simulink model "volo_radio_controller"  (Simulink 8.0)
settings: Solver=ode45  SolverMode=SingleTasking  StartTime=0.0  StopTime=1000  RelTol=1e-3
InitFcn:
  | volo_radio_controller_init
values from neighbouring files (symbols this model uses):
  cFI = fi(cMult, 1, 13, 11)    [volo_radio_controller_init.m]
  gFI = fi(gain, 1, 13, 11)    [volo_radio_controller_init.m]
  sFI = fi(sMult, 1, 13, 11)    [volo_radio_controller_init.m]
undefined symbols (not defined in the file or in its folder): gcbh, xlBlockLoadCallback, xlGetNormalizedPeriod, xlipgetpartsetting
libraries: xbsIndex_r4 x380, xbsEDKLib_r4 x1
(part 1 of 5)
settings Model: Creator=naren  LastModifiedBy=rng
settings DataIOCC: SignalLoggingSaveFormat=ModelDataLogs
settings DebuggingCC: FcnCallInpInsideContextMsg=UseLocalSettings
settings GRTTargetCC: CombineOutputUpdateFcns=off  GRTInterface=on

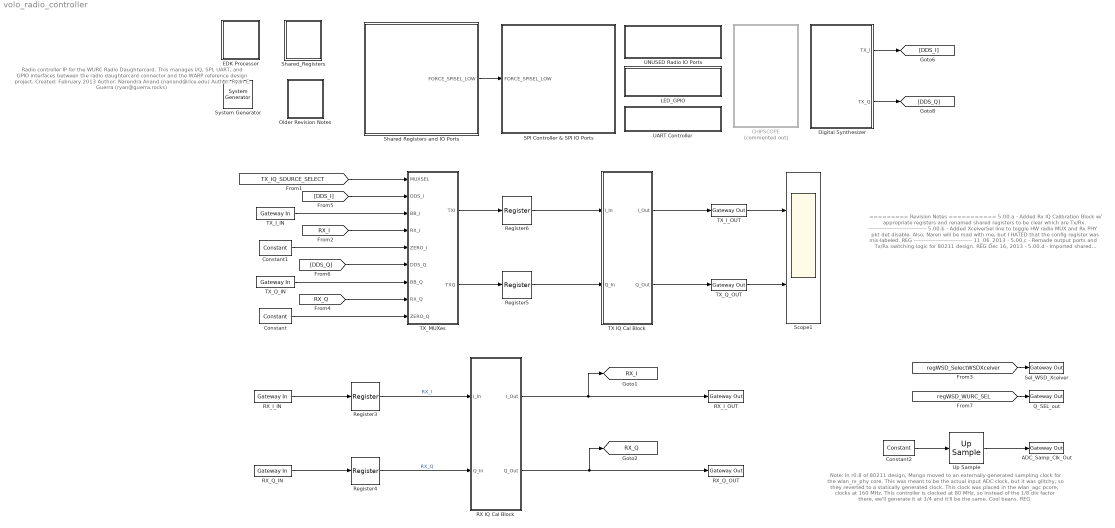
== system volo_radio_controller ==
  note: Note: in r0.8 of 80211 design, Mango moved to an externally-generated sampling clock for the wlan_rx_phy
      | core. This was meant to be the actual input ADC clock, but it was glitchy, so they reverted to a statically generated clock.
      | This clock was placed in the wlan_agc pcore, clocks at 160 MHz. This controller is clocked at 80 MHz, so instead of the 1/8
      | div factor there, we'll generate it at 1/4 and it'll be the same. Cool beans. REG
  note: Radio controller IP for the WURC Radio Daughtercard.
      | This manages I/Q, SPI, UART, and GPIO interfaces
      | between the radio daughtercard connector and the
      | WARP reference design project.
      |
      | Created: February 2013
      | Author: Narendra Anand (nanand@rice.edu)
      | Author: Ryan E. Guerra (ryan@guerra.rocks)
  note: ========= Revision Notes ===========
      | 5.00.a - Added Rx IQ Calibration Block w/ appropriate registers and renamed shared
      | registers to be clear which are Tx/Rx.
      | -----------------------------------
      | 5.00.b - Added XceiverSel line to toggle HW radio MUX and Rx PHY pkt det disable.
      | Also, Naren will be mad with me, but I HATED that the config register was mis-labeled. REG
      | -----------------------------------
      | 11_06_2013 - 5.00.c - Remade output ports and Tx/Rx switching logic for 80211 design. REG
      | Dec 16, 2013 - 5.00.d - Imported shared registers from Tx/Rx FIR to save on AXI Slave slots REG
      | Jan 15, 2014 - 5.00.e - Removed filter stuff and cleaned up for 802.11 Rev0.7 REG
      | Jan 17, 2014 - 5.00.f - removed extra ports to avoid confusion. Better to add than take away REG
      | Feb 13, 2014 - 5.00.g - added ADC_SAMP_CLK_OUT port for compatibility with rev 0.8 design REG
      | April 22, 2014 - 5.00.h - Changed DDS synthesizer tp fixed Sysgen core for better frequency response
      | AND removed the corresponding DDS registers (phaseInc and ddsOutputReset) NA
      | April 29, 2014 - 5.00.i - Previous version had some EDK register screwup, fixed now.  NA
      | April 30, 2014 - 5.00.j - Added taylor series correction setting to dds compiler, maximized DSP
      | utilization and set goal to speed.
      | May 23, 2014 - 5.08.k - WOW! EDK Processor was creating duplicate register offset addresses.
      | This was the problem that was borking everything. NOTE: it is still not fixed, but we have gone and
      | hand-edited the MPD file with unique, non-overlapping offsets for the To/From registers. REG
      | May 23, 2014 - 5.08.m - EDK Processor didn't synthesize 5 registers. Reinitialized Processor and
      | am trying again. REG
      | May 26, 2014 - 5.08.q - Diagnosed error with unchecked register read-back. REG
      | Nov 21, 2014 - 2.08.r - Regened for Naren for SysGen 14.4. REG
      | Jan 02, 2015 - 2.08.s - Added latency to cast at the end of IQ Cal Blocks. REG
      | Jan 18, 2015 - 2.08.t - Added 2-bit radio sel lines to general options register,
      | added output Q_Sel_out. REG
      | Jan 19, 2015 - 2.08.u - added pipeline registers to the SPI output lines to avoid logn routes. REG
  " System Generator" : xbsIndex_r4/ System Generator  Tag=genX  xilinxfamily=virtex6  part=xc6vcx240t  speed=-2  package=ff1156  synthesis_tool=XST  clock_wrapper=Clock Enables  directory=./volo_radio_pcore_generated_pcores  proj_type=Project Navigator  Synth_file=XST Defaults  Impl_file=ISE Defaults  testbench=off  simulink_period=1  sysclk_period=10  dcm_input_clock_period=10  incr_netlist=off  trim_vbits=Everywhere in SubSystem  dbl_ovrd=According to Block Masks  core_generation=According to Block Masks  run_coregen=off  deprecated_control=off  eval_field=0  block_type=sysgen
  ADC_Samp_Clk_Out : xbsIndex_r4/Gateway Out  inherit_from_input=off  hdl_port=on  timing_constraint=None  locs_specified=off  LOCs={}  UseAsDAC=off  DACChannel='1'  block_type=gatewayout
      settings: infoedit="Gateway out block.  Converts Xilinx fixed-point or floating-point type inputs into ouputs of type Simulink integer, single, double, or fixed point.<br><br>Hardware notes:  In hardware these blocks become top level output ports or are discarded, depending on how they are configured."  xl_area=[0 0 0 0 12 0 0]
  CHIPSCOPE : Subsystem  Commented=on
  Constant : xbsIndex_r4/Constant  const=0  gui_display_data_type=Fixed-point  arith_type=Signed (2's comp)  n_bits=12  bin_pt=11  preci_type=Single  exp_width=8  frac_width=24  explicit_period=off  period=1  equ=P=C  opselect=C  inp2=PCIN>>17  opr=+  inp1=P  carry=CIN  dbl_ovrd=off  block_type=constant
  Constant1 : xbsIndex_r4/Constant  const=0  gui_display_data_type=Fixed-point  arith_type=Signed (2's comp)  n_bits=12  bin_pt=11  preci_type=Single  exp_width=8  frac_width=24  explicit_period=off  period=1  equ=P=C  opselect=C  inp2=PCIN>>17  opr=+  inp1=P  carry=CIN  dbl_ovrd=off  block_type=constant
  Constant2 : xbsIndex_r4/Constant  const=1  gui_display_data_type=Boolean  arith_type=Boolean  n_bits=16  bin_pt=14  preci_type=Single  exp_width=8  frac_width=24  explicit_period=on  period=4  equ=P=C  opselect=C  inp2=PCIN>>17  opr=+  inp1=P  carry=CIN  dbl_ovrd=off  block_type=constant
  Digital Synthesizer : Subsystem
  EDK Processor : Subsystem  LoadFcn=xlBlockLoadCallback(gcbh);  mask(Xilinx EDK Processor Block){mode=EDK pcore generation, xmp=, MemVisToProc=<qt bgcolor="#FFFFFF"><div><img src="E:/Xilinx_ISE_14_4/14.4/ISE_DS/ISE/sysgen/data/images/registerplus.gif"> &lt;&lt;VOLO_CONTROLLER_CONFIG_R&gt;&gt;<br></div><div><img src="E:/Xilinx_ISE_14_4/14.4/ISE_DS/ISE/sysgen/data/images/registerplus.gif"> &lt;&lt;VOLO_SPI_SRCSEL&gt;&gt;<br></div><div><img src="E:/Xilinx_ISE_14_4/14.4/ISE_DS/ISE/sysgen/data/images/registerplus.gif"> &lt;&lt;VOLO_SPI_GO&gt;&gt;<br></div><div><img src="E:/Xilinx_ISE_14_4/14.4/ISE_DS/ISE/sysgen/data/images/registerplus.gif"> &lt;&lt;VOLO_RX_COS_MULT&gt;&gt;<br></div><div><img src="E:/Xilinx_ISE_14_4/14.4/ISE_DS/ISE/sysgen/data/images/registerplus.gif"> &lt;&lt;VOLO_RX_GAIN_MULT&gt;&gt;<br></div><div><img src="E:/Xilinx_ISE_14_4/14.4/ISE_DS/ISE/sysgen/data/images/registerplus.gif"> &lt;&lt;VOLO_SPI_TXDAT&gt;&gt;<br></div><div><img src="E:/Xilinx_ISE_14_4/14.4/ISE_DS/ISE/sysgen/data/images/registerplus.gif"> &lt;&lt;VOLO_RX_SIN_MULT&gt;&gt;<br></div><div><img src="E:/Xilinx_ISE_14_4/14.4/ISE_DS/ISE/sysgen/data/images/registerplus.gif"> &lt;&lt;VOLO_TX_COS_MULT&gt;&gt;<br></div><div><img src="E:/Xilinx_ISE_14_4/14.4/ISE_DS/ISE/sysgen/data/images/registerplus.gif"> &lt;&lt;VOLO_TX_GAIN_MULT&gt;&gt;<br></div><div><img src="E:/Xilinx_ISE_14_4/14.4/ISE_DS/ISE/sysgen/data/images/registerplus.gif"> &lt;&lt;VOLO_TX_SIN_MULT&gt;&gt;<br></div><div><img src="E:/Xilinx_ISE_14_4/14.4/ISE_DS/ISE/sysgen/data/images/registerplus.gif"> &lt;&lt;WSD_SPIWAITDELAYCOUNT&gt;&gt;<br></div><div><img src="E:/Xilinx_ISE_14_4/14.4/ISE_DS/ISE/sysgen/data/images/registerplus.gif"> &lt;&lt;WSD_RXSWITCHINGDELAYCOUNT&gt;&gt;<br></div><div><img src="E:/Xilinx_ISE_14_4/14.4/ISE_DS/ISE/sysgen/data/images/registerplus.gif"> &lt;&lt;WSD_SWITCHINGDELAYCOUNT&gt;&gt;<br></div><div><img src="E:/Xilinx_ISE_14_4/14.4/ISE_DS/ISE/sysgen/data/images/registerplus.gif"> &lt;&lt;VOLO_ADAPTER_GPIO&gt;&gt;<br></div><div><img src="E:/Xilinx_ISE_14_4/14.4/ISE_DS/ISE/sysgen/data/images/registerplus.gif"> &lt;&lt;VOLO_LED&gt;&gt;<br></div><div><img src="E:/Xilinx_ISE_14_4/14.4/ISE_DS/ISE/sysgen/data/images/registerplus.gif"> &lt;&lt;VOLO_SPI_RST&gt;&gt;<br></div><div><img src="E:/Xilinx_ISE_14_4/14.4/ISE_DS/ISE/sysgen/data/images/registerplus.gif"> &lt;&lt;VOLO_SETTINGS&gt;&gt;<br></div><div><img src="E:/Xilinx_ISE_14_4/14.4/ISE_DS/ISE/sysgen/data/images/registerplus.gif"> &lt;&lt;VOLO_SPI_RXDAT&gt;&gt;<br></div><div><img src="E:/Xilinx_ISE_14_4/14.4/ISE_DS/ISE/sysgen/data/images/registerplus.gif"> &lt;&lt;VOLO_SPI_DONE&gt;&gt;<br></div></qt>, AvailableMemories=<empty>, portInterfaceTable={'exposed'=>[],'portdir'=>[],'portname'=>[],'shortname'=>[]}, bus_type_sgadvanced=, bus_type=AXI, baseaddr=0x80000000, baseaddr_lock_sgadvanced=, baseaddr_lock=off, dual_clock_sgadvanced=, dual_clock=on, reg_readback_sgadvanced=, reg_readback=on, ucf_file=, inheritDeviceType_sgadvanced=, inheritDeviceType=off, elf_file=, codebug_sgadvanced=, codebug=on, clock_name=plb, internalPortList={}, resetPolarity=0, memxtable={'mladdr'=>[0.00000000000000000,1.00000000000000000,2.00000000000000000,3.00000000000000000,4.00000000000000000,5.00000000000000000,6.00000000000000000,7.00000000000000000,8.00000000000000000,9.00000000000000000,10.00000000000000000,11.00000000000000000,12.00000000000000000,13.00000000000000000,14.00000000000000000,15.00000000000000000,16.00000000000000000,0.00000000000000000,1.00000000000000000],'mlist'=>['volo_radio_controller/Shared_Registers/From Register5','volo_radio_controller/Shared_Registers/From Register4','volo_radio_controller/Shared_Registers/From Register3','volo_radio_controller/Shared_Registers/From Register21','volo_radio_controller/Shared_Registers/From Register20','volo_radio_controller/Shared_Registers/From Register2','volo_radio_controller/Shared_Registers/From Register19','volo_radio_controller/Shared_Registers/From Register18','volo_radio_controller/Shared_Registers/From Register17','volo_radio_controller/Shared_Registers/From Register16','volo_radio_controller/Shared_Registers/From Register15','volo_radio_controller/Shared_Registers/From Register14','volo_radio_controller/Shared_Registers/From Register13','volo_radio_controller/Shared_Registers/From Register12','volo_radio_controller/Shared_Registers/From Register11','volo_radio_controller/Shared_Registers/From Register1','volo_radio_controller/Shared_Registers/From Register','volo_radio_controller/SPI Controller & SPI IO Ports/To Register1','volo_radio_controller/SPI Controller & SPI IO Ports/To Register'],'mlname'=>['\'VOLO_CONTROLLER_CONFIG_R\'','\'VOLO_SPI_SRCSEL\'','\'VOLO_SPI_GO\'','\'VOLO_RX_COS_MULT\'','\'VOLO_RX_GAIN_MULT\'','\'VOLO_SPI_TXDAT\'','\'VOLO_RX_SIN_MULT\'','\'VOLO_TX_COS_MULT\'','\'VOLO_TX_GAIN_MULT\'','\'VOLO_TX_SIN_MULT\'','\'WSD_SPIWAITDELAYCOUNT\'','\'WSD_RXSWITCHINGDELAYCOUNT\'','\'WSD_SWITCHINGDELAYCOUNT\'','\'VOLO_ADAPTER_GPIO\'','\'VOLO_LED\'','\'VOLO_SPI_RST\'','\'VOLO_SETTINGS\'','\'VOLO_SPI_RXDAT\'','\'VOLO_SPI_DONE\''],'mlstate'=>[0.00000000000000000,0.00000000000000000,0.00000000000000000,0.00000000000000000,0.00000000000000000,0.00000000000000000,0.00000000000000000,0.00000000000000000,0.00000000000000000,0.00000000000000000,0.00000000000000000,0.00000000000000000,0.00000000000000000,0.00000000000000000,0.00000000000000000,0.00000000000000000,0.00000000000000000,0.00000000000000000,0.00000000000000000]}, procinfo={}, memmapdirty=off, blockname=, xpsintstyle=default, has_advanced_control=0, sggui_pos=-1471,122,939,804, block_type=edkprocessor, block_version=2.7, sg_icon_stat=62,64,-1,-1,white,blue,0,07734,right,,[ ],[ ], sg_mask_display=|, sg_list_contents={'table'=>{'AvailableMemories'=>'popup(<empty>)'}}, sg_blockgui_xml=}
      mask sg_mask_display=|
      | fprintf('','COMMENT: begin icon graphics');
      | patch([0 62 62 0 0 ],[0 0 64 64 0 ],[0.77 0.82 0.91 ]);
      | plot([0 62 62 0 0 ],[0 0 64 64 0 ]);
      | patch([13.2 24.76 32.76 40.76 48.76 32.76 21.2 13.2 ],[40.88 40.88 48.88 40.88 48.88 48.88 48.88 40.88 ],[1 1 1 ]);
      | patch([21.2 32.76 24.76 13.2 21.2 ],[32.88 32.88 40.88 40.88 32.88 ],[0.931 0.946 0.973 ]);
      | patch([13.2 24.76 32.76 21.2 13.2 ],[24.88 24.88 32.88 32.88 24.88 ],[1 1 1 ]);
      | patch([21.2 48.76 40.76 32.76 24.76 13.2 21.2 ],[16.88 16.88 24.88 16.88 24.88 24.88 16.88 ],[0.931 0.946 0.973 ]);
      | fprintf('','COMMENT: end icon graphics');
      | fprintf('','COMMENT: begin icon text');
      | fprintf('','COMMENT: end icon text');
      mask prompts: mode "Configure Processor for"; xmp "XPS Project"; MemVisToProc ""; AvailableMemories "Available Memories"; portInterfaceTable ""; bus_type_sgadvanced ""; bus_type "Bus Type"; baseaddr "Base Address"; baseaddr_lock_sgadvanced ""; baseaddr_lock "Lock"; dual_clock_sgadvanced ""; dual_clock "Dual Clocks"; reg_readback_sgadvanced ""; reg_readback "Register Read-Back"; ucf_file "Constraint File"; inheritDeviceType_sgadvanced ""; inheritDeviceType "Inherit Device Type"; elf_file "Initial Program"; codebug_sgadvanced ""; codebug "Enable Co-Debug with Xilinx SDK (Beta)"; clock_name ""; internalPortList ""; resetPolarity ""; memxtable ""; procinfo ""; memmapdirty ""; blockname ""; xpsintstyle ""; has_advanced_control ""; sggui_pos ""; block_type ""; block_version ""; sg_icon_stat ""; sg_mask_display ""; sg_list_contents ""; sg_blockgui_xml ""
      mask help: Xilinx EDK Processor
      mask init:
      | try
      |   tmp_gcb = gcb;
      |   tmp_gcbh = gcbh;
      |   if (strcmp('SysGenIndex',get_param(bdroot(tmp_gcbh),'tag')) && ~isempty(regexp(bdroot(tmp_gcb), '^xbs', 'once')))
      |     return;
      |   end;
      |   xlMungeMaskParams;
      | 
      |   block_type='edkprocessor';
      | 
      |   serialized_declarations = '{''block_type''=>''String''}';
      |   xledkprocessor_init();
      |   ptable_ = xlblockprep(get_param(tmp_gcb, 'MaskWSVariables'));
      |   try
      |     xlBlockMoveCallback(tmp_gcbh);
      |   catch 
      |      clear global xl_updateicon_recursion_guard;
      |   end;
      | catch
      |   global dbgsysgen;
      |   if(~isempty(dbgsysgen) && dbgsysgen)
      |     e = regexprep(lasterr, '\n', '\nError: ');
      |     disp(['Error: While running MaskInit code on block ' tmp_gcb ': ' e]);
      |     error(e);
      |   end
      | end
      settings: CopyFcn=xlProcBlockCopyCallback(gcbh);xlBlockMoveCallback(gcbh);  DeleteFcn=xlDestroyGui(gcbh);  ModelCloseFcn=xlDestroyGui(gcbh);  PreSaveFcn=xlBlockPreSaveCallback(gcbh);  PostSaveFcn=xlBlockPostSaveCallback(gcbh);  DestroyFcn=xlDestroyGui(gcbh);  OpenFcn=bh=gcbh;xlProcBlockCallbacks('populatesharedmemorylistbox',bh);xlOpenGui(bh, 'edkprocessor_gui.xml', @xlProcBlockEnablement, @xlProcBlockAction);  CloseFcn=xlDestroyGui(gcbh);  MoveFcn=xlBlockMoveCallback(gcbh);
      mask Help: eval('');xlDoc('-book','sysgen','-topic','EDK_Processor');
      mask TypeOptions mode: EDK pcore generation | HDL netlisting
      mask TypeOptions bus_type: AXI | PLB
      mask Display:
      | fprintf('','COMMENT: begin icon graphics');
      | patch([0 62 62 0 0 ],[0 0 64 64 0 ],[0.77 0.82 0.91 ]);
      | plot([0 62 62 0 0 ],[0 0 64 64 0 ]);
      | patch([13.2 24.76 32.76 40.76 48.76 32.76 21.2 13.2 ],[40.88 40.88 48.88 40.88 48.88 48.88 48.88 40.88 ],[1 1 1 ]);
      | patch([21.2 32.76 24.76 13.2 21.2 ],[32.88 32.88 40.88 40.88 32.88 ],[0.931 0.946 0.973 ]);
      | patch([13.2 24.76 32.76 21.2 13.2 ],[24.88 24.88 32.88 32.88 24.88 ],[1 1 1 ]);
      | patch([21.2 48.76 40.76 32.76 24.76 13.2 21.2 ],[16.88 16.88 24.88 16.88 24.88 24.88 16.88 ],[0.931 0.946 0.973 ]);
      | fprintf('','COMMENT: end icon graphics');
      | fprintf('','COMMENT: begin icon text');
      | disp('');
      | 
      | fprintf('','COMMENT: end icon text');
  LED_GPIO : Subsystem
  Older Revision Notes : Subsystem
  Q_SEL_out : xbsIndex_r4/Gateway Out  inherit_from_input=off  hdl_port=on  timing_constraint=None  locs_specified=off  LOCs={}  UseAsDAC=off  DACChannel='1'  block_type=gatewayout
      settings: infoedit="Gateway out block.  Converts Xilinx fixed-point or floating-point type inputs into ouputs of type Simulink integer, single, double, or fixed point.<br><br>Hardware notes:  In hardware these blocks become top level output ports or are discarded, depending on how they are configured."  xl_area=[0 0 0 0 12 0 0]
  RX IQ Cal Block : Subsystem
  RX_I_IN : xbsIndex_r4/Gateway In  gui_display_data_type=Fixed-point  arith_type="Signed  (2's comp)"  n_bits=12  bin_pt=11  preci_type=Single  exp_width=8  frac_width=24  quantization="Round  (unbiased: +/- Inf)"  overflow=Saturate  period=2  dbl_ovrd=off  timing_constraint=None  locs_specified=off  LOCs={}  UseAsADC=off  ADCChannel='1'  inherit_from_input=off  hdl_port=on  block_type=gatewayin
      settings: xl_area=[0 0 0 0 12 0 0]
  RX_I_OUT : xbsIndex_r4/Gateway Out  inherit_from_input=off  hdl_port=on  timing_constraint=None  locs_specified=off  LOCs={}  UseAsDAC=off  DACChannel='1'  block_type=gatewayout
      settings: infoedit="Gateway out block.  Converts Xilinx fixed-point or floating-point type inputs into ouputs of type Simulink integer, single, double, or fixed point.<br><br>Hardware notes:  In hardware these blocks become top level output ports or are discarded, depending on how they are configured."  xl_area=[0 0 0 0 1 0 0]
  RX_Q_IN : xbsIndex_r4/Gateway In  gui_display_data_type=Fixed-point  arith_type="Signed  (2's comp)"  n_bits=12  bin_pt=11  preci_type=Single  exp_width=8  frac_width=24  quantization="Round  (unbiased: +/- Inf)"  overflow=Saturate  period=2  dbl_ovrd=off  timing_constraint=None  locs_specified=off  LOCs={}  UseAsADC=off  ADCChannel='1'  inherit_from_input=off  hdl_port=on  block_type=gatewayin
      settings: xl_area=[0 0 0 0 12 0 0]
  RX_Q_OUT : xbsIndex_r4/Gateway Out  inherit_from_input=off  hdl_port=on  timing_constraint=None  locs_specified=off  LOCs={}  UseAsDAC=off  DACChannel='1'  block_type=gatewayout
      settings: infoedit="Gateway out block.  Converts Xilinx fixed-point or floating-point type inputs into ouputs of type Simulink integer, single, double, or fixed point.<br><br>Hardware notes:  In hardware these blocks become top level output ports or are discarded, depending on how they are configured."  xl_area=[0 0 0 0 1 0 0]
  Register3 : xbsIndex_r4/Register  init=0  rst=off  en=off  dbl_ovrd=off  block_type=register
      settings: xl_area=[6 12 0 0 0 0 0]  block_version=8.2
  Register4 : xbsIndex_r4/Register  init=0  rst=off  en=off  dbl_ovrd=off  block_type=register
      settings: xl_area=[6 12 0 0 0 0 0]  block_version=8.2
  Register5 : xbsIndex_r4/Register  init=0  rst=off  en=off  dbl_ovrd=off  block_type=register
      settings: xl_area=[1 1 0 0 0 0 0]  block_version=8.2
  Register6 : xbsIndex_r4/Register  init=1  rst=off  en=off  dbl_ovrd=off  block_type=register
      settings: xl_area=[1 1 0 0 0 0 0]  block_version=8.2
  SPI Controller & SPI IO Ports : Subsystem
  Scope1 : Scope  NumInputPorts=2
      settings: YMin=-5~-5  YMax=5~5  SaveName=ScopeData4
  Sel_WSD_Xceiver : xbsIndex_r4/Gateway Out  inherit_from_input=off  hdl_port=on  timing_constraint=None  locs_specified=off  LOCs={}  UseAsDAC=off  DACChannel='1'  block_type=gatewayout
      settings: infoedit="Gateway out block.  Converts Xilinx fixed-point or floating-point type inputs into ouputs of type Simulink integer, single, double, or fixed point.<br><br>Hardware notes:  In hardware these blocks become top level output ports or are discarded, depending on how they are configured."  xl_area=[0 0 0 0 12 0 0]
  Shared Registers and IO Ports : Subsystem
  Shared_Registers : Subsystem
  TX IQ Cal Block : Subsystem
  TX_I_IN : xbsIndex_r4/Gateway In  gui_display_data_type=Fixed-point  arith_type="Signed  (2's comp)"  n_bits=12  bin_pt=11  preci_type=Single  exp_width=8  frac_width=24  quantization="Round  (unbiased: +/- Inf)"  overflow=Saturate  period=2  dbl_ovrd=off  timing_constraint=None  locs_specified=off  LOCs={}  UseAsADC=off  ADCChannel='1'  inherit_from_input=off  hdl_port=on  block_type=gatewayin
      settings: xl_area=[0 0 0 0 1 0 0]
  TX_I_OUT : xbsIndex_r4/Gateway Out  inherit_from_input=off  hdl_port=on  timing_constraint=None  locs_specified=off  LOCs={}  UseAsDAC=off  DACChannel='1'  block_type=gatewayout
      settings: infoedit="Gateway out block.  Converts Xilinx fixed-point or floating-point type inputs into ouputs of type Simulink integer, single, double, or fixed point.<br><br>Hardware notes:  In hardware these blocks become top level output ports or are discarded, depending on how they are configured."  xl_area=[0 0 0 0 1 0 0]
  TX_MUXes : Subsystem
  TX_Q_IN : xbsIndex_r4/Gateway In  gui_display_data_type=Fixed-point  arith_type="Signed  (2's comp)"  n_bits=12  bin_pt=11  preci_type=Single  exp_width=8  frac_width=24  quantization="Round  (unbiased: +/- Inf)"  overflow=Saturate  period=2  dbl_ovrd=off  timing_constraint=None  locs_specified=off  LOCs={}  UseAsADC=off  ADCChannel='1'  inherit_from_input=off  hdl_port=on  block_type=gatewayin
      settings: xl_area=[0 0 0 0 1 0 0]
  TX_Q_OUT : xbsIndex_r4/Gateway Out  inherit_from_input=off  hdl_port=on  timing_constraint=None  locs_specified=off  LOCs={}  UseAsDAC=off  DACChannel='1'  block_type=gatewayout
      settings: infoedit="Gateway out block.  Converts Xilinx fixed-point or floating-point type inputs into ouputs of type Simulink integer, single, double, or fixed point.<br><br>Hardware notes:  In hardware these blocks become top level output ports or are discarded, depending on how they are configured."  xl_area=[0 0 0 0 12 0 0]
  UART Controller : Subsystem
  UNUSED Radio IO Ports : Subsystem
  Up Sample : xbsIndex_r4/Up Sample  sample_ratio=4  copy_samples=off  en=off  latency=0  dbl_ovrd=off  block_type=usamp
  tag scope: RX_I=global, RX_Q=global
  wires:
  RX IQ Cal Block/1(I_Out) -> RX_I_OUT/1, [RX_I]
  TX_MUXes/1(TXI) -> Register6/1
  TX_MUXes/2(TXQ) -> Register5/1
  RX_I_IN/1 -> Register3/1
  RX_Q_IN/1 -> Register4/1
  TX_I_OUT/1 -> Scope1/1
  TX_Q_OUT/1 -> Scope1/2
  TX IQ Cal Block/1(I_Out) -> TX_I_OUT/1
  TX IQ Cal Block/2(Q_Out) -> TX_Q_OUT/1
  [TX_IQ_SOURCE_SELECT] -> TX_MUXes/1(MUXSEL)
  Digital Synthesizer/1(TX_I) -> [DDS_I]
  Digital Synthesizer/2(TX_Q) -> [DDS_Q]
  [DDS_I] -> TX_MUXes/2(DDS_I)
  [DDS_Q] -> TX_MUXes/6(DDS_Q)
  [RX_I] -> TX_MUXes/4(RX_I)
  [RX_Q] -> TX_MUXes/8(RX_Q)
  TX_I_IN/1 -> TX_MUXes/3(BB_I)
  TX_Q_IN/1 -> TX_MUXes/7(BB_Q)
  Register5/1 -> TX IQ Cal Block/2(Q_In)
  Register6/1 -> TX IQ Cal Block/1(I_In)
  Constant1/1 -> TX_MUXes/5(ZERO_I)
  Constant/1 -> TX_MUXes/9(ZERO_Q)
  Shared Registers and IO Ports/1(FORCE_SPISEL_LOW) -> SPI Controller & SPI IO Ports/1(FORCE_SPISEL_LOW)
  RX IQ Cal Block/2(Q_Out) -> [RX_Q], RX_Q_OUT/1
  Register3/1 -> RX IQ Cal Block/1(I_In)  "RX_I"
  Register4/1 -> RX IQ Cal Block/2(Q_In)  "RX_Q"
  [regWSD_SelectWSDXceiver] -> Sel_WSD_Xceiver/1
  Constant2/1 -> Up Sample/1
  Up Sample/1 -> ADC_Samp_Clk_Out/1
  [regWSD_WURC_SEL] -> Q_SEL_out/1

== system volo_radio_controller/CHIPSCOPE ==
  ChipScope : xbsIndex_r4/ChipScope  Commented=on  num_trig_ports=4  current_port=0  show_trig_port=0  match_units=1  match_type=Basic with edges  data_is_trigger=on  num_data_ports=2  data_depth=65536  SRL16s=on  add_bufg=on  match_type_t0=2  match_type_t1=1  match_type_t2=1  match_type_t3=1  match_type_t4=1  match_type_t5=1  match_type_t6=1  match_type_t7=1  match_type_t8=1  match_type_t9=1  match_type_t10=1  match_type_t11=1  match_type_t12=1  match_type_t13=1  match_type_t14=1  match_type_t15=1  match_units_t0=1  match_units_t1=1  match_units_t2=1  match_units_t3=1  match_units_t4=1  match_units_t5=1  match_units_t6=1  match_units_t7=1  match_units_t8=1  match_units_t9=1  match_units_t10=1  match_units_t11=1  match_units_t12=1  match_units_t13=1  match_units_t14=1  match_units_t15=1  dbl_ovrd=0  user_scan_chain=USER1  block_type=chipscope
      settings: infoedit="Enables run-time debugging and verification of signals by inserting ChipScope Pro ICON and ILA cores.<br><br>  Restrictions: <br>Only one ChipScope core can be instantiated in a System Generator design. A design or subsystem containing a ChipScope block must have at least one output port."
  Disregard Subsystem : xbsIndex_r4/Disregard Subsystem  Tag=discardX  block_type=disregard
  From1 : From  Commented=on  GotoTag=RX_CLKOUT  TagVisibility=global
  From2 : From  Commented=on  GotoTag=RX_IQSEL  TagVisibility=global
  From4 : From  Commented=on  GotoTag=RX_I  TagVisibility=global
  From5 : From  Commented=on  GotoTag=RX_Q  TagVisibility=global
  wires:
  From4/1 -> ChipScope/3  "RX_I"
  From5/1 -> ChipScope/4  "RX_Q"
  From1/1 -> ChipScope/1
  From2/1 -> ChipScope/2

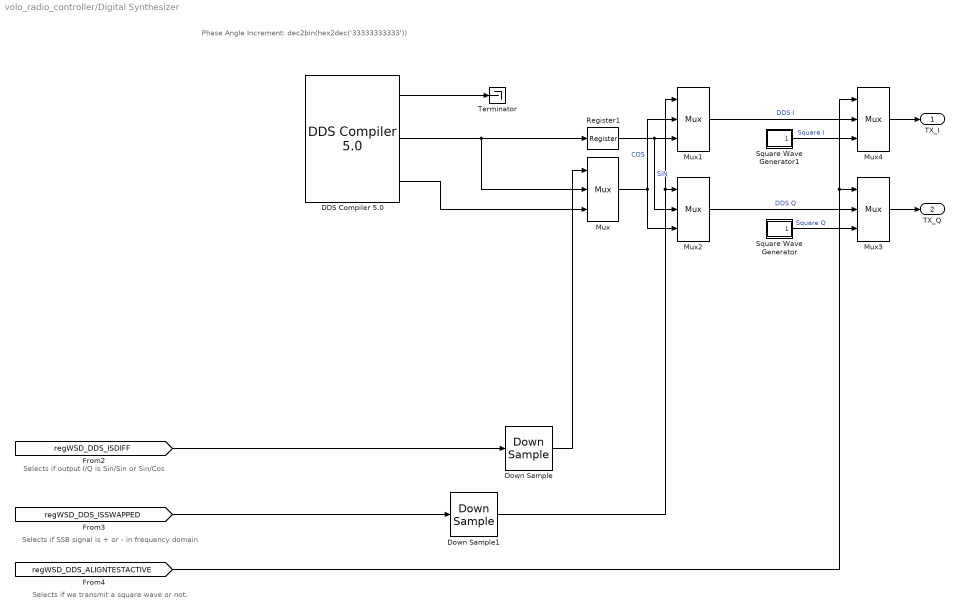
== system volo_radio_controller/Digital Synthesizer ==
  note: Phase Angle Increment:
      | dec2bin(hex2dec('33333333333'))
  note: Selects if SSB signal is + or - in frequency domain
  note: Selects if output I/Q is Sin/Sin or Sin/Cos
  note: Selects if we transmit a square wave or not.
  "DDS Compiler 5.0 " : xbsIndex_r4/DDS Compiler 5.0   partspresent=Phase_Generator_and_SIN_COS_LUT  dds_clock_rate=80  channels=1  parameter_entry=Hardware_Parameters  spurious_free_dynamic_range=36  frequency_resolution=0.4  noise_shaping=Taylor_Series_Corrected  phase_width=48  output_width=12  output_selection=Sine_and_Cosine  negative_sine=off  negative_cosine=off  amplitude_mode=Full_Range  memory_type=Auto  optimization_goal=Speed  dsp48_use=Maximal  latency_configuration=Auto  latency=8  has_phase_out=off  has_aclken=off  has_aresetn=off  explicit_period=off  period=1  data_has_tlast=Not_Required  has_tready=off  s_phase_has_tuser=Not_Required  m_data_has_tuser=Not_Required  m_phase_has_tuser=Not_Required  s_phase_tuser_width=1  s_config_sync_mode=On_Vector  phase_increment=Fixed  output_frequency1=0  output_frequency2=0  output_frequency3=0  output_frequency4=0  output_frequency5=0  output_frequency6=0  output_frequency7=0  output_frequency8=0  output_frequency9=0  output_frequency10=0  output_frequency11=0  output_frequency12=0  output_frequency13=0  output_frequency14=0  output_frequency15=0  output_frequency16=0  pinc1=dds_generator_phase_inc_binary  pinc2='0'  pinc3='0'  pinc4='0'  pinc5='0'  pinc6='0'  pinc7='0'  pinc8='0'  pinc9='0'  pinc10='0'  pinc11='0'  pinc12='0'  pinc13='0'  pinc14='0'  pinc15='0'  pinc16='0'  phase_offset=None  phase_offset_angles1=0  phase_offset_angles2=0  phase_offset_angles3=0  phase_offset_angles4=0  phase_offset_angles5=0  phase_offset_angles6=0  phase_offset_angles7=0  phase_offset_angles8=0  phase_offset_angles9=0  phase_offset_angles10=0  phase_offset_angles11=0  phase_offset_angles12=0  phase_offset_angles13=0  phase_offset_angles14=0  phase_offset_angles15=0  phase_offset_angles16=0  poff1='0'  poff2='0'  poff3='0'  poff4='0'  poff5='0'  poff6='0'  poff7='0'  poff8='0'  poff9='0'  poff10='0'  poff11='0'  poff12='0'  poff13='0'  poff14='0'  poff15='0'  poff16='0'  trim_axipin_name=on  por_mode=false  gui_behaviour=Sysgen  ip_name=DDS Compiler  ip_version=5.0  dsptool_ready=true  wrapper_available=true  port_translation_map={ 'aclken' => 'en', 'aresetn' => 'rst' }  ipcore_xco_need_fpga_part=true  ipcore_fpga_part=xlipgetpartsetting(gcb, {'virtex6', 'xc6vlx75t', '-3', 'ff784'})  ipcore_usecache=true  ipcore_useipmodelcache=true  ipcore_verbose=false  block_type=dds_compiler_v5_0
  Down Sample : xbsIndex_r4/Down Sample  sample_ratio=2  sample_phase="Last Value of Frame  (most efficient)"  en=off  latency=1  dbl_ovrd=off  block_type=dsamp
      settings: xl_area=[1 1 0 0 0 0 0]
  Down Sample1 : xbsIndex_r4/Down Sample  sample_ratio=2  sample_phase="Last Value of Frame  (most efficient)"  en=off  latency=1  dbl_ovrd=off  block_type=dsamp
      settings: xl_area=[1 1 0 0 0 0 0]
  Mux{,1..4} (5 alike) : xbsIndex_r4/Mux  inputs=2  en=off  latency=1  precision=Full  arith_type=Unsigned  n_bits=16  bin_pt=14  quantization=Truncate  overflow=Wrap  dbl_ovrd=off  block_type=mux
      settings: xl_area=[6 12 0 12 0 0 0]
  Register1 : xbsIndex_r4/Register  init=0  rst=off  en=off  dbl_ovrd=off  block_type=register
      settings: xl_area=[6 12 0 0 0 0 0]  block_version=8.2
  Square Wave Generator : Subsystem
  Square Wave Generator1 : Subsystem
  Terminator : Terminator
  TX_I : Outport
  TX_Q : Outport  Port=2
  wires:
  Mux/1 -> Mux2/3, Mux1/2  "COS"
  [regWSD_DDS_ISDIFF] -> Down Sample/1
  Down Sample/1 -> Mux/1
  Mux2/1 -> Mux3/2  "DDS Q"
  Mux1/1 -> Mux4/2  "DDS I"
  Register1/1 -> Mux1/3, Mux2/2  "SIN"
  [regWSD_DDS_ISSWAPPED] -> Down Sample1/1
  Down Sample1/1 -> Mux1/1, Mux2/1
  Mux3/1 -> TX_Q/1
  Mux4/1 -> TX_I/1
  [regWSD_DDS_ALIGNTESTACTIVE] -> Mux4/1, Mux3/1
  Square Wave Generator1/1(Out) -> Mux4/3  "Square I"
  Square Wave Generator/1(Out) -> Mux3/3  "Square Q"
  "DDS Compiler 5.0 "/2 -> Mux/2, Register1/1
  "DDS Compiler 5.0 "/3 -> Mux/3
  "DDS Compiler 5.0 "/1 -> Terminator/1
